simulink model "dc_bus_pi_vs_lstm"  (R2025b)
settings: Solver=FixedStepDiscrete  StartTime=0  StopTime=6  FixedStep=0.01  RelTol=1e-3
settings Model: Creator=riyaj  LastModifiedBy=riyaj

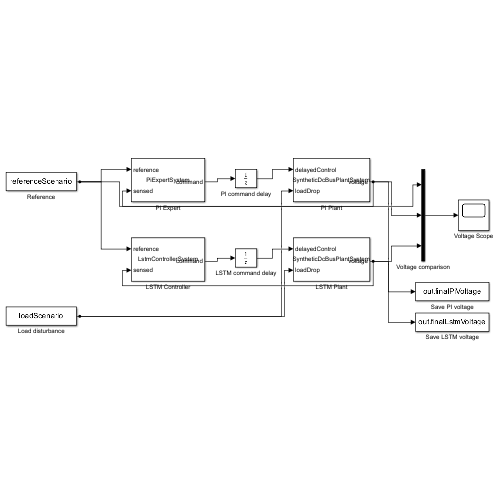
[thumbnail: Simulink's stored preview of the top-level diagram]
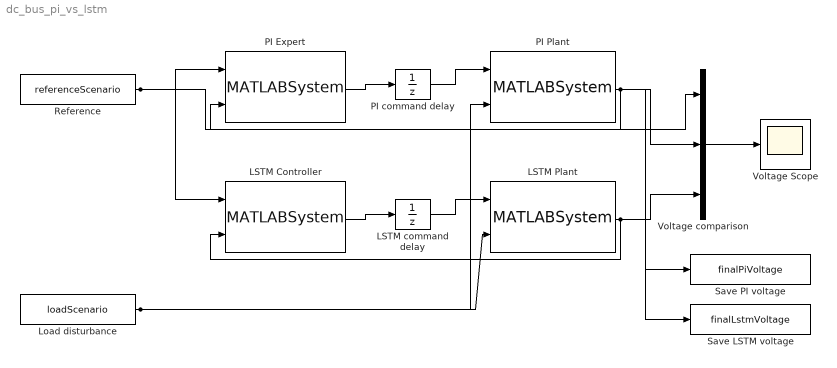
== system dc_bus_pi_vs_lstm ==
  LSTM Controller : MATLABSystem  System=LstmControllerSystem  SimulateUsing=Interpreted execution
      mask Type: LstmControllerSystem
  LSTM Plant : MATLABSystem  System=SyntheticDcBusPlantSystem  Tau=0.35  ControlGain=2.5  SampleTime=0.01  NominalVoltage=300  InitialVoltage=298  SimulateUsing=Interpreted execution
      mask Type: SyntheticDcBusPlantSystem
  LSTM command delay : UnitDelay  SampleTime=0.01  HasFrameUpgradeWarning=on
  Load disturbance : FromWorkspace  VariableName=loadScenario
  PI Expert : MATLABSystem  System=PiExpertSystem  Kp=0.65  Ki=2.5  SampleTime=0.01  LowerLimit=-10  UpperLimit=10  SimulateUsing=Interpreted execution
      mask Type: PiExpertSystem
  PI Plant : MATLABSystem  System=SyntheticDcBusPlantSystem  Tau=0.35  ControlGain=2.5  SampleTime=0.01  NominalVoltage=300  InitialVoltage=298  SimulateUsing=Interpreted execution
      mask Type: SyntheticDcBusPlantSystem
  PI command delay : UnitDelay  SampleTime=0.01  HasFrameUpgradeWarning=on
  Reference : FromWorkspace  VariableName=referenceScenario
  Save LSTM voltage : ToWorkspace  VariableName=finalLstmVoltage  SaveFormat=Timeseries  SampleTime=-1
  Save PI voltage : ToWorkspace  VariableName=finalPiVoltage  SaveFormat=Timeseries  SampleTime=-1
  Voltage Scope : Scope
  Voltage comparison : Mux  Inputs=3
  wires:
  Reference/1 -> PI Expert/1, LSTM Controller/1, Voltage comparison/1
  PI Expert/1 -> PI command delay/1
  LSTM Controller/1 -> LSTM command delay/1
  PI command delay/1 -> PI Plant/1
  LSTM command delay/1 -> LSTM Plant/1
  Load disturbance/1 -> PI Plant/2, LSTM Plant/2
  PI Plant/1 -> PI Expert/2, Voltage comparison/2, Save PI voltage/1
  LSTM Plant/1 -> LSTM Controller/2, Voltage comparison/3, Save LSTM voltage/1
  Voltage comparison/1 -> Voltage Scope/1
